simulink model "BBBC_4"  (R2022b)
settings: Solver=VariableStepAuto  StartTime=0.0  StopTime=3  RelTol=1e-3
undefined symbols (not defined in the file): dct, dEv, Ev, sigbuilder_block
libraries: simulink x5, spsMosfetLib x4, spsSeriesRLCBranchLib x4, spsCurrentMeasurementLib x2, spsVoltageMeasurementLib x2, spsGroundLib x1, spsControlledVoltageSourceLib x1, spspowerguiLib x1
settings Model: Creator=Dopechuro  LastModifiedBy=Dopechuro

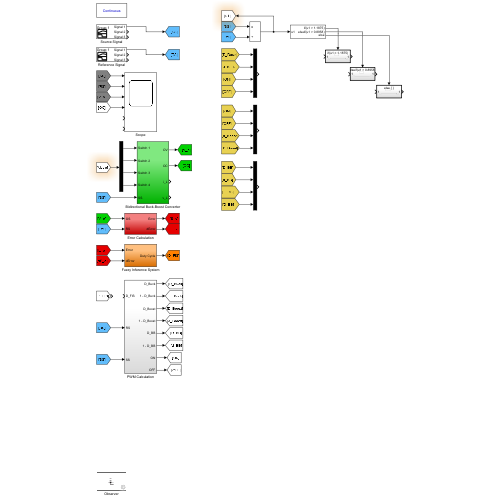
[thumbnail: Simulink's stored preview of the top-level diagram]
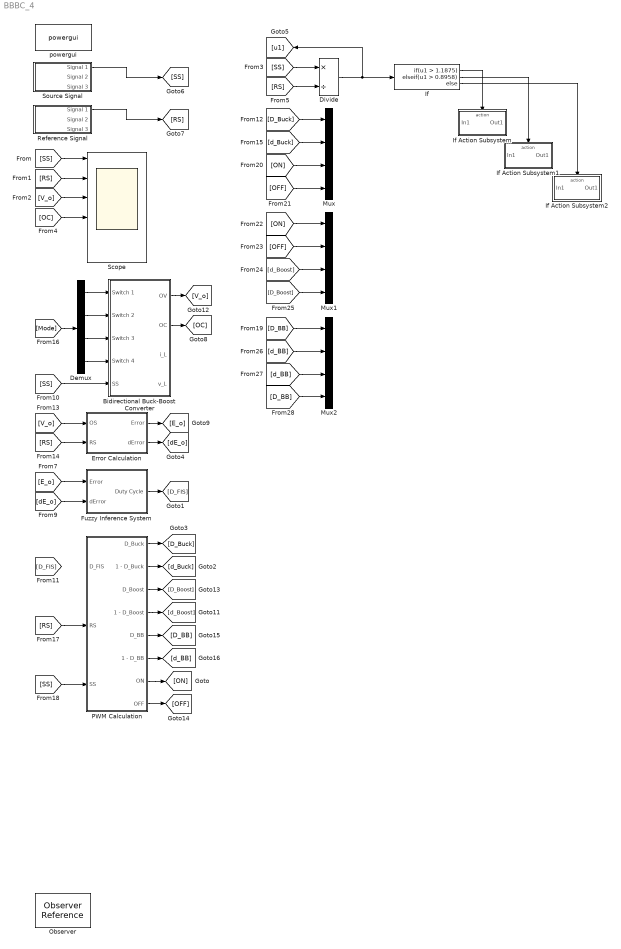
== system BBBC_4 ==
  Bidirectional Buck-Boost Converter : Subsystem
  Demux : Demux
  Divide : Product  Inputs=*/
  Error Calculation : Subsystem
  Fuzzy Inference System : Subsystem
  If : If  IfExpression=u1 > 1.1875  ElseIfExpressions=u1 > 0.8958
  If Action Subsystem : Subsystem  TreatAsAtomicUnit=on
  If Action Subsystem1 : Subsystem  TreatAsAtomicUnit=on
  If Action Subsystem2 : Subsystem  TreatAsAtomicUnit=on
  Mux : Mux
  Mux1 : Mux
  Mux2 : Mux
  Observer : ObserverReference  ObserverModelName=BBBC_4_Observer1
  PWM Calculation : Subsystem
  Reference Signal : Subsystem  Tag=STV Subsys  LoadFcn=sigbuilder_block('load');  StartFcn=sigbuilder_block('start');  StopFcn=sigbuilder_block('stop');  ClipboardFcn=sigbuilder_block('clipboard');  mask(Sigbuilder block){tuvar=[0:10]}
      mask help: Simulink:masks:SigbuilderBlock_MD
      mask init:
      | if ~strcmp(get_param(bdroot(gcbh),'SimulationStatus'),'stopped') tuvar = sigbuilder_block('maskInit'); end
      settings: CopyFcn=sigbuilder_block('copy');  DeleteFcn=sigbuilder_block('delete');  ModelCloseFcn=sigbuilder_block('modelClose');  PreSaveFcn=sigbuilder_block('preSave');  PauseFcn=sigbuilder_block('pause');  ContinueFcn=sigbuilder_block('continue');  NameChangeFcn=sigbuilder_block('namechange');  OpenFcn=sigbuilder_block('open',[530.25 309.75 550.5 399.75 ]);  CloseFcn=sigbuilder_block('close');
      mask Display: plot(0, 0, 100, 100,[2, 2, 32, 32, 2], [68, 8, 8, 68, 68],[32, 2], [38, 38], [32, 19, 2],[53, 60, 44], [32, 17, 17, 2],[16, 16, 31, 31]);txt = getActiveGroup(gcbh);text(2, 100, txt,'verticalAlignment', 'top');
  Scope : Scope  NumInputPorts=6
  Source Signal : Subsystem  Tag=STV Subsys  LoadFcn=sigbuilder_block('load');  StartFcn=sigbuilder_block('start');  StopFcn=sigbuilder_block('stop');  ClipboardFcn=sigbuilder_block('clipboard');  mask(Sigbuilder block){tuvar=[0:10]}
      mask help: Simulink:masks:SigbuilderBlock_MD
      mask init:
      | if ~strcmp(get_param(bdroot(gcbh),'SimulationStatus'),'stopped') tuvar = sigbuilder_block('maskInit'); end
      settings: CopyFcn=sigbuilder_block('copy');  DeleteFcn=sigbuilder_block('delete');  ModelCloseFcn=sigbuilder_block('modelClose');  PreSaveFcn=sigbuilder_block('preSave');  PauseFcn=sigbuilder_block('pause');  ContinueFcn=sigbuilder_block('continue');  NameChangeFcn=sigbuilder_block('namechange');  OpenFcn=sigbuilder_block('open',[395.25 256.5 550.5 399.75 ]);  CloseFcn=sigbuilder_block('close');
      mask Display: plot(0, 0, 100, 100,[2, 2, 32, 32, 2], [68, 8, 8, 68, 68],[32, 2], [38, 38], [32, 19, 2],[53, 60, 44], [32, 17, 17, 2],[16, 16, 31, 31]);txt = getActiveGroup(gcbh);text(2, 100, txt,'verticalAlignment', 'top');
  powergui : spspowerguiLib/powergui  Priority=1  SimulationMode=Continuous  SampleTime=50e-6  frequency=60  Iterations=50  frequencyindice=0  Pbase=100e6  ErrMax=1e-4  UnitsV=kV  UnitsW=MW  buscounter=0  FunctionMessages=off  echomessages=off  EnableUseOfTLC=off  CurrentSourceSwitches=off  DisableSnubberDevices=off  DisableRonSwitches=off  DisableVfSwitches=off  DisplayEquations=off  AutomaticDiscreteSolvers=off  SolverType=Tustin/Backward Euler (TBE)  Interpol=off  ExternalGateDelay=off  methode=off  Ts=100  x0status=blocks  SPID=on  SwTol=0  HookPort=off  NonlinearTolerance=1e-4  nMaxIteration=100  ContinueOnMaxIteration=off  RestoreLinks=warning  ResistiveCurrentMeasurement=off  Frange=[0:2:500]  Ylog=off  Xlog=on  ShowGrid=off  save=off  variable=ZData  structure=0  ZoomFFT=off  StartTime=0.0  cycles=1  DisplayStyle=1  fundamental=60  FreqAxis=off  MaxFrequency=1000  frequencyindicesteady=1  RmsSteady=1  display=off
  wires:
  [RS] -> Scope/2
  [V_o] -> Scope/3
  [V_o] -> Error Calculation/1(OS)
  [RS] -> Error Calculation/2(RS)
  Error Calculation/1(Error) -> [E_o]
  Error Calculation/2(dError) -> [dE_o]
  [SS] -> Scope/1
  [SS] -> Bidirectional Buck-Boost Converter/5(SS)
  Bidirectional Buck-Boost Converter/1(OV) -> [V_o]
  [E_o] -> Fuzzy Inference System/1(Error)
  [dE_o] -> Fuzzy Inference System/2(dError)
  Fuzzy Inference System/1(Duty Cycle) -> [D_FIS]
  [RS] -> Divide/2
  [SS] -> Divide/1
  [D_Buck] -> Mux/1
  [d_Buck] -> Mux/2
  [ON] -> Mux/3
  [OFF] -> Mux/4
  [ON] -> Mux1/1
  [OFF] -> Mux1/2
  [d_Boost] -> Mux1/3
  [D_Boost] -> Mux1/4
  [Mode] -> Demux/1
  Demux/2 -> Bidirectional Buck-Boost Converter/2(Switch 2)
  Demux/1 -> Bidirectional Buck-Boost Converter/1(Switch 1)
  [RS] -> PWM Calculation/2(RS)
  [SS] -> PWM Calculation/3(SS)
  Demux/4 -> Bidirectional Buck-Boost Converter/4(Switch 4)
  Demux/3 -> Bidirectional Buck-Boost Converter/3(Switch 3)
  PWM Calculation/2(1 - D_Buck) -> [d_Buck]
  PWM Calculation/1(D_Buck) -> [D_Buck]
  PWM Calculation/4(1 - D_Boost) -> [d_Boost]
  PWM Calculation/7(ON) -> [ON]
  PWM Calculation/8(OFF) -> [OFF]
  PWM Calculation/3(D_Boost) -> [D_Boost]
  PWM Calculation/5(D_BB) -> [D_BB]
  PWM Calculation/6(1 - D_BB) -> [d_BB]
  [D_BB] -> Mux2/4
  [D_BB] -> Mux2/1
  [d_BB] -> Mux2/3
  [d_BB] -> Mux2/2
  Reference Signal/1(Signal 1) -> [RS]
  Source Signal/1(Signal 1) -> [SS]
  Bidirectional Buck-Boost Converter/2(OC) -> [OC]
  [OC] -> Scope/4
  Divide/1 -> If/1, [u1]
  If/1 -> If Action Subsystem/Action
  If/2 -> If Action Subsystem1/Action
  If/3 -> If Action Subsystem2/Action

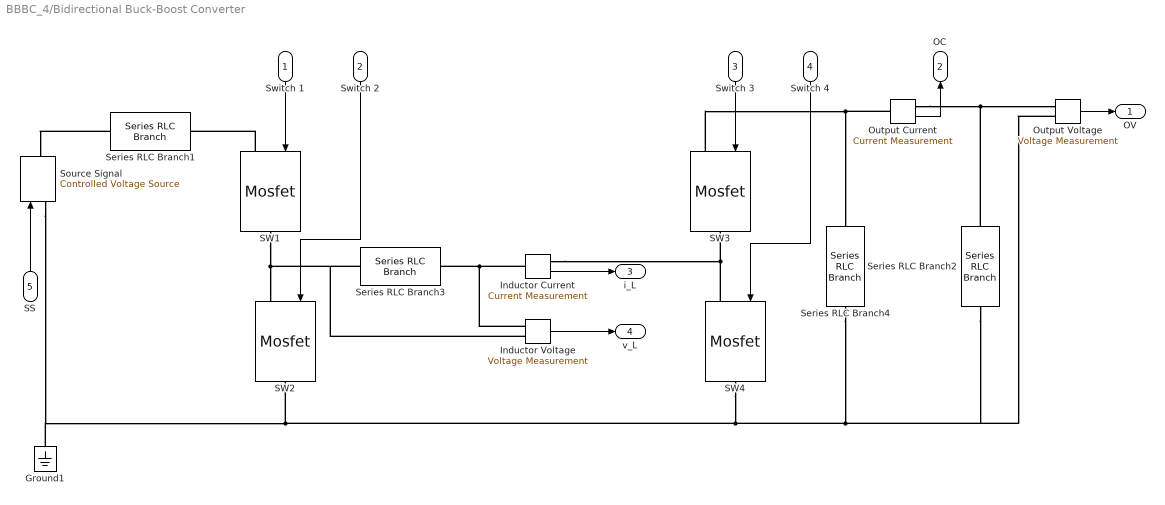
== system BBBC_4/Bidirectional Buck-Boost Converter ==
  Switch 1 : Inport
  Switch 2 : Inport  Port=2
  Switch 3 : Inport  Port=3
  Switch 4 : Inport  Port=4
  SS : Inport  Port=5
  Ground1 : spsGroundLib/Ground  LConnTagsString=a
  Inductor Current : spsCurrentMeasurementLib/Current Measurement  PhasorSimulation=off  OutputType=Complex  PSBequivalent=0
  Inductor Voltage : spsVoltageMeasurementLib/Voltage Measurement  PhasorSimulation=off  OutputType=Complex  PSBequivalent=0
  Output Current : spsCurrentMeasurementLib/Current Measurement  PhasorSimulation=off  OutputType=Complex  PSBequivalent=0
  Output Voltage : spsVoltageMeasurementLib/Voltage Measurement  PhasorSimulation=off  OutputType=Complex  PSBequivalent=0
  SW{1..4} (4 alike) : spsMosfetLib/Mosfet  Ron=0.1  Lon=0  Rd=0.01  Vfd=0  IC=0  Rs=1e5  Cs=inf  Measurements=off
  Series RLC Branch1 : spsSeriesRLCBranchLib/Series RLC Branch  LConnTagsString=__new0  RConnTagsString=__new0  BranchType=R  Resistance=0.1  Inductance=1e-3  SetiL0=off  InitialCurrent=0  Capacitance=1e-6  Setx0=off  InitialVoltage=0  Measurements=None
  Series RLC Branch2 : spsSeriesRLCBranchLib/Series RLC Branch  LConnTagsString=__new0  RConnTagsString=__new0  BranchType=R  Resistance=24  Inductance=1e-3  SetiL0=off  InitialCurrent=0  Capacitance=1000e-6  Setx0=off  InitialVoltage=0  Measurements=None
  Series RLC Branch3 : spsSeriesRLCBranchLib/Series RLC Branch  LConnTagsString=__new0  RConnTagsString=__new0  BranchType=RL  Resistance=0.1  Inductance=0.434e-3  SetiL0=off  InitialCurrent=0  Capacitance=1e-6  Setx0=off  InitialVoltage=0  Measurements=None
  Series RLC Branch4 : spsSeriesRLCBranchLib/Series RLC Branch  LConnTagsString=__new0  RConnTagsString=__new0  BranchType=RC  Resistance=0.01  Inductance=1e-3  SetiL0=off  InitialCurrent=0  Capacitance=10.6e-6  Setx0=off  InitialVoltage=0  Measurements=None
  Source Signal : spsControlledVoltageSourceLib/Controlled Voltage Source  Initialize=off  Source_Type=DC  Amplitude=0  Phase=0  Frequency=0  Measurements=None
  OV : Outport
  OC : Outport  Port=2
  i_L : Outport  Port=3
  v_L : Outport  Port=4
  wires:
  Switch 1/1 -> SW1/1
  Switch 3/1 -> SW3/1
  Switch 2/1 -> SW2/1
  SS/1 -> Source Signal/1
  Switch 4/1 -> SW4/1
  Inductor Current/1 -> i_L/1
  Output Voltage/1 -> OV/1
  Inductor Voltage/1 -> v_L/1
  Output Current/1 -> OC/1
  connections:
  SW1/LConn1 -- Series RLC Branch1/RConn1
  Inductor Current/LConn1 -- Inductor Voltage/LConn2 -- Series RLC Branch3/RConn1
  SW4/LConn1 -- Inductor Current/RConn1 -- SW3/RConn1
  SW4/RConn1 -- Output Voltage/LConn2 -- Series RLC Branch2/RConn1 -- Series RLC Branch4/RConn1 -- Source Signal/LConn1 -- Ground1/LConn1 -- SW2/RConn1
  SW1/RConn1 -- Inductor Voltage/LConn1 -- Series RLC Branch3/LConn1 -- SW2/LConn1
  Series RLC Branch1/LConn1 -- Source Signal/RConn1
  Output Current/RConn1 -- Output Voltage/LConn1 -- Series RLC Branch2/LConn1
  SW3/LConn1 -- Output Current/LConn1 -- Series RLC Branch4/LConn1

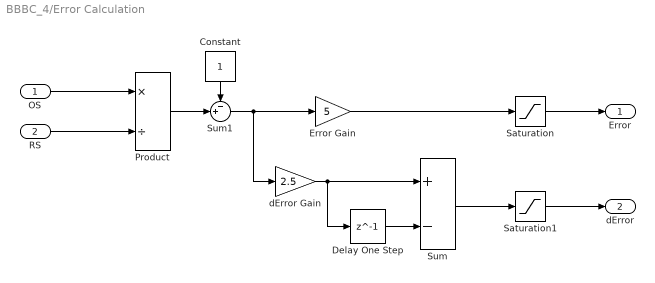
== system BBBC_4/Error Calculation ==
  OS : Inport
  RS : Inport  Port=2
  Constant : Constant
  Delay One Step : Delay  DelayLength=1
  Error Gain : Gain  Gain=5
  Product : Product  Inputs=*/
  Saturation : Saturate  UpperLimit=1  LowerLimit=-1
  Saturation1 : Saturate  UpperLimit=1  LowerLimit=-1
  Sum : Sum  Inputs=+-
  Sum1 : Sum  Inputs=-+|
  dError Gain : Gain  Gain=2.5
  Error : Outport
  dError : Outport  Port=2
  wires:
  Sum1/1 -> dError Gain/1, Error Gain/1
  dError Gain/1 -> Sum/1, Delay One Step/1
  Error Gain/1 -> Saturation/1
  Constant/1 -> Sum1/1
  Delay One Step/1 -> Sum/2
  Product/1 -> Sum1/2
  Sum/1 -> Saturation1/1
  OS/1 -> Product/1
  RS/1 -> Product/2
  Saturation/1 -> Error/1
  Saturation1/1 -> dError/1

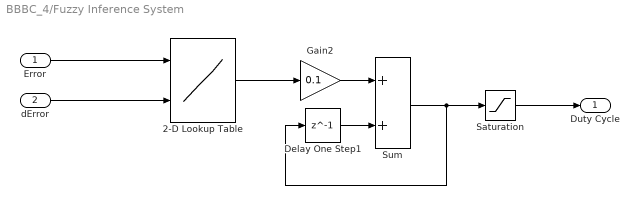
== system BBBC_4/Fuzzy Inference System ==
  Error : Inport
  dError : Inport  Port=2
  2-D Lookup Table : Lookup_n-D  LookupTableObject=''  BreakpointsForDimension1=Ev  BreakpointsForDimension2=dEv  BreakpointsForDimension1FirstPoint=10  BreakpointsForDimension2FirstPoint=10  BreakpointsForDimension1Spacing=12  BreakpointsForDimension2Spacing=12  IndexSearchMethod=Evenly spaced points  Table=dct  InterpMethod=Nearest  DiagnosticForOutOfRangeInput=Warning  InternalRulePriority=Speed  OutDataTypeStr=Inherit: Inherit from 'Table data'  RndMeth=Simplest
      settings: InputPortMap=u0,u1
  Delay One Step1 : Delay  DelayLength=1
  Gain2 : Gain  Gain=0.1
  Saturation : Saturate  UpperLimit=0.9  LowerLimit=-0.9
  Sum : Sum
  Duty Cycle : Outport
  wires:
  Delay One Step1/1 -> Sum/2
  Sum/1 -> Saturation/1, Delay One Step1/1
  Gain2/1 -> Sum/1
  2-D Lookup Table/1 -> Gain2/1
  Saturation/1 -> Duty Cycle/1
  Error/1 -> 2-D Lookup Table/1
  dError/1 -> 2-D Lookup Table/2

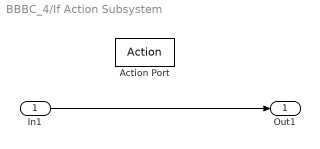
== system BBBC_4/If Action Subsystem ==
  In1 : Inport
  Action Port : ActionPort  ActionPortLabel=if(u1 > 1.1875)
  Out1 : Outport
  wires:
  In1/1 -> Out1/1

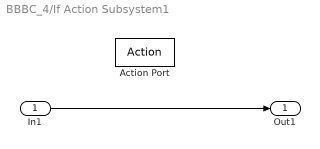
== system BBBC_4/If Action Subsystem1 ==
  In1 : Inport
  Action Port : ActionPort  ActionPortLabel=elseif(u1 > 0.8958)
  Out1 : Outport
  wires:
  In1/1 -> Out1/1

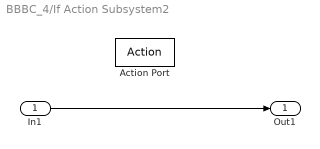
== system BBBC_4/If Action Subsystem2 ==
  In1 : Inport
  Action Port : ActionPort  ActionPortLabel=else
  Out1 : Outport
  wires:
  In1/1 -> Out1/1

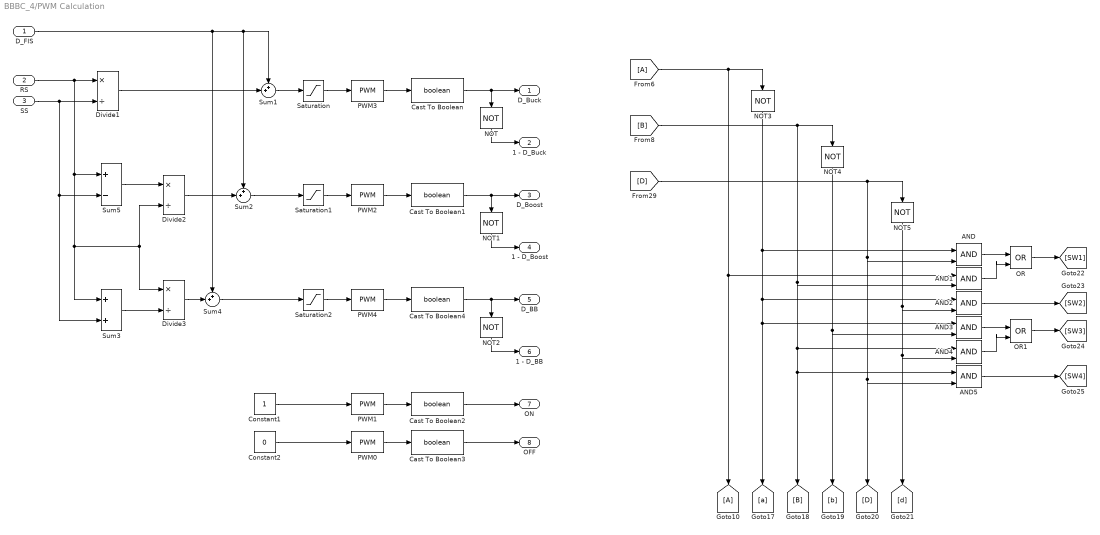
== system BBBC_4/PWM Calculation ==
  D_FIS : Inport
  RS : Inport  Port=2
  SS : Inport  Port=3
  AND{,1..5} (6 alike) : Logic  IconShape=distinctive  AllPortsSameDT=off  OutDataTypeStr=boolean
  Cast To Boolean{,1..4} (5 alike) : DataTypeConversion  OutDataTypeStr=boolean  SaturateOnIntegerOverflow=off  RndMeth=Floor
  Constant1 : Constant
  Constant2 : Constant  Value=0
  Divide1 : Product  Inputs=*/
  Divide2 : Product  Inputs=*/
  Divide3 : Product  Inputs=*/
  From6 : From
  Goto10 : Goto
  NOT{,1..5} (6 alike) : Logic  Operator=NOT  IconShape=distinctive  AllPortsSameDT=off  OutDataTypeStr=boolean
  OR : Logic  Operator=OR  IconShape=distinctive  AllPortsSameDT=off  OutDataTypeStr=boolean
  OR1 : Logic  Operator=OR  IconShape=distinctive  AllPortsSameDT=off  OutDataTypeStr=boolean
  PWM{0..4} (5 alike) : simulink/Discontinuities/PWM  DisableCoverage=on  Period=1/1e4  InitialDelay=0  DisallowZeroDutyCycle=off  RunAtFixedTimeIntervals=off  SampleTime=0.1
  Saturation : Saturate  UpperLimit=0.85  LowerLimit=0.1
  Saturation1 : Saturate  UpperLimit=0.85  LowerLimit=0.1
  Saturation2 : Saturate  UpperLimit=0.85  LowerLimit=0.1
  Sum1 : Sum  Inputs=++|
  Sum2 : Sum  Inputs=++|
  Sum3 : Sum
  Sum4 : Sum  Inputs=++|
  Sum5 : Sum  Inputs=+-
  D_Buck : Outport
  1 - D_Buck : Outport  Port=2
  D_Boost : Outport  Port=3
  1 - D_Boost : Outport  Port=4
  D_BB : Outport  Port=5
  1 - D_BB : Outport  Port=6
  ON : Outport  Port=7
  OFF : Outport  Port=8
  wires:
  Divide1/1 -> Sum1/2
  RS/1 -> Divide1/1, Sum5/1, Divide2/2, Divide3/1, Sum3/1
  SS/1 -> Divide1/2, Sum5/2, Sum3/2
  NOT/1 -> 1 - D_Buck/1
  Sum2/1 -> Saturation1/1
  PWM2/1 -> Cast To Boolean1/1
  NOT1/1 -> 1 - D_Boost/1
  PWM0/1 -> Cast To Boolean3/1
  PWM1/1 -> Cast To Boolean2/1
  PWM3/1 -> Cast To Boolean/1
  Sum1/1 -> Saturation/1
  Constant2/1 -> PWM0/1
  Constant1/1 -> PWM1/1
  D_FIS/1 -> Sum1/1, Sum2/1, Sum4/1
  Cast To Boolean/1 -> NOT/1, D_Buck/1
  Cast To Boolean1/1 -> NOT1/1, D_Boost/1
  Cast To Boolean2/1 -> ON/1
  Cast To Boolean3/1 -> OFF/1
  Saturation/1 -> PWM3/1
  Saturation1/1 -> PWM2/1
  Saturation2/1 -> PWM4/1
  PWM4/1 -> Cast To Boolean4/1
  Cast To Boolean4/1 -> NOT2/1, D_BB/1
  NOT2/1 -> 1 - D_BB/1
  Sum3/1 -> Divide3/2
  Divide3/1 -> Sum4/2
  Sum4/1 -> Saturation2/1
  Divide2/1 -> Sum2/2
  Sum5/1 -> Divide2/1
  AND2/1 -> [SW2]
  AND/1 -> OR/1
  NOT3/1 -> AND/1, AND2/1, AND3/1, [a]
  NOT5/1 -> [d], AND4/2, AND2/2
  [B] -> AND1/2, AND4/1, AND5/1, [B], NOT4/1
  AND1/1 -> OR/2
  AND5/1 -> [SW4]
  OR1/1 -> [SW3]
  From6/1 -> AND1/1, Goto10/1, NOT3/1
  [D] -> NOT5/1, AND5/2, [D], AND/2
  NOT4/1 -> [b], AND3/2
  AND3/1 -> OR1/1
  OR/1 -> [SW1]
  AND4/1 -> OR1/2

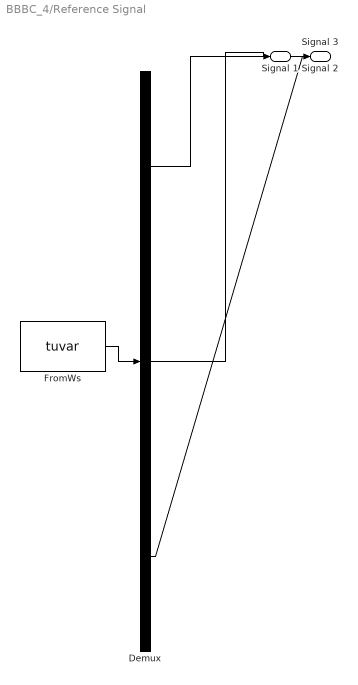
== system BBBC_4/Reference Signal ==
  Demux : Demux  Tag=STV Demux  Outputs=3
      settings: DisplayOption=none
  FromWs : FromWorkspace  Tag=STV FromWs  VariableName=tuvar
      SigBuilderData=|
      | common.afterFinalStr = 'Extrapolate'
      | common.sampleTime = 0
      | dataSet.timeRange = [0 3]
      | dataSet.name = 'Group 1'
      | sbobj.Groups.Name = 'Group 1'
      | sbobj.Groups.Signals(1).Name = 'Signal 1'
      | sbobj.Groups.Signals(1).XData = [0 3]
      | sbobj.Groups.Signals(1).YData = [5 5]
      | sbobj.Groups.Signals(2).Name = 'Signal 2'
      | sbobj.Groups.Signals(2).XData = [0 1.5 1.5 3]
      | sbobj.Groups.Signals(2).YData = [5 5 2.6 2.6]
      | sbobj.Groups.Signals(3).Name = 'Signal 3'
      | sbobj.Groups.Signals(3).XData = [0 0.1 0.2 0.3 0.4 0.5 0.6 0.7 0.8 0.9 1 1.1 1.2 1.3 1.4 1.5 1.6 1.7 1.8 1.9 2 2.1 2.2 2.3 2.4 2.5 2.6 2.7 2.8 2.9 3]
      | sbobj.Groups.Signals(3).YData = [3.36966244158 3.38350881651 3.27562848596 3.32156700864 3.18341560685 3.18520472211 3.3104874716 3.37222540322 3.55854912526 3.23331093293 3.31873310246 3.29175055746 3.10669770821 3.25610338461 3.12053211585 3.38403755298 3.21119679177 3.31000928331 3.245547107 3.33035207946 3.23996734379 3.34899653212 3.37393631236 3.4711887783 3.28058764642 3.08616447306 3.21604112527 3.4354594328 3.19278447116 3.39609538697 3.31240498]
      | sbobj.Groups.TimeRange = [0 3]
  Signal 1 : Outport  Tag=STV Outport
  Signal 2 : Outport  Tag=STV Outport  Port=2
  Signal 3 : Outport  Tag=STV Outport  Port=3
  wires:
  FromWs/1 -> Demux/1
  Demux/1 -> Signal 1/1
  Demux/2 -> Signal 2/1
  Demux/3 -> Signal 3/1

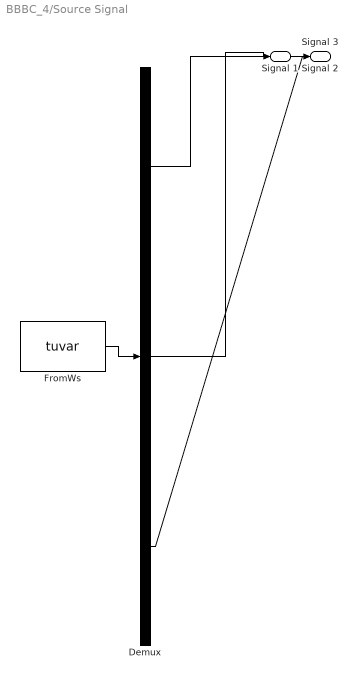
== system BBBC_4/Source Signal ==
  Demux : Demux  Tag=STV Demux  Outputs=3
      settings: DisplayOption=none
  FromWs : FromWorkspace  Tag=STV FromWs  VariableName=tuvar
      SigBuilderData=|
      | common.afterFinalStr = 'Extrapolate'
      | common.sampleTime = 0
      | dataSet.timeRange = [0 3]
      | dataSet.name = 'Group 1'
      | sbobj.Groups.Name = 'Group 1'
      | sbobj.Groups.Signals(1).Name = 'Signal 1'
      | sbobj.Groups.Signals(1).XData = [0 3]
      | sbobj.Groups.Signals(1).YData = [12 12]
      | sbobj.Groups.Signals(2).Name = 'Signal 2'
      | sbobj.Groups.Signals(2).XData = [0 0.1 0.2 0.3 0.4 0.5 0.6 0.7 0.8 0.9 1 1.1 1.2 1.3 1.4 1.5 1.6 1.7 1.8 1.9 2 2.1 2.2 2.3 2.4 2.5 2.6 2.7 2.8 2.9 3]
      | sbobj.Groups.Signals(2).YData = [3.17858829564 3.18864992585 3.29931506719 3.45326303083 3.22303340862 3.33713788128 3.27744155977 3.41173561388 3.19109357049 3.30325574642 3.35525270211 3.41006102179 3.45442118955 3.30859311332 3.15084096894 3.22576981627 3.19384182667 3.5350457224 3.23843981185 3.37480767837 3.28075814894 3.38886104254 3.22351507634 3.15977310307 3.15776240749 3.34881939099 3.28226248434 3.28039465122 3.44193101506 3.3291584374 3.31978110535]
      | sbobj.Groups.Signals(3).Name = 'Signal 3'
      | sbobj.Groups.Signals(3).XData = [0 0.1 0.2 0.3 0.4 0.5 0.6 0.7 0.8 0.9 1 1.1 1.2 1.3 1.4 1.5 1.6 1.7 1.8 1.9 2 2.1 2.2 2.3 2.4 2.5 2.6 2.7 2.8 2.9 3]
      | sbobj.Groups.Signals(3).YData = [3.31774301561 3.36051820548 3.22545805359 3.32845171957 3.31051925292 3.25684628622 3.28569146326 3.3113066074 3.41808709901 3.39139142199 3.25545373097 3.40015247439 3.32393833942 3.29791918918 3.32358651583 3.29323612008 3.29590323651 3.34916002106 3.34649813816 3.34676734964 3.32215940541 3.26015293155 3.32366887549 3.35379776454 3.31613349442 3.33414486933 3.3239872094 3.28998644948 3.30969775841 3.27401966748 3.32931705585]
      | sbobj.Groups.TimeRange = [0 3]
  Signal 1 : Outport  Tag=STV Outport
  Signal 2 : Outport  Tag=STV Outport  Port=2
  Signal 3 : Outport  Tag=STV Outport  Port=3
  wires:
  FromWs/1 -> Demux/1
  Demux/1 -> Signal 1/1
  Demux/2 -> Signal 2/1
  Demux/3 -> Signal 3/1
